simulink model "pwm1"  (R2012b)
settings: Solver=ode45  StartTime=0.0  StopTime=0.1  FixedStep=0.4e-4  RelTol=1e-3
libraries: Tools x5
settings Model: Creator=h3now  LastModifiedBy=h3now

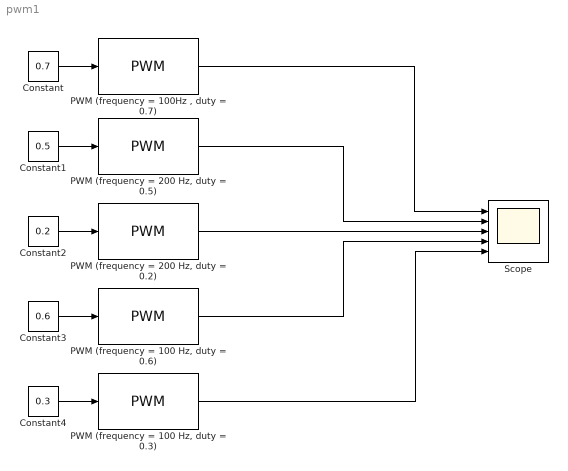
== system pwm1 ==
  Constant : Constant  Value=0.7
  Constant1 : Constant  Value=0.5
  Constant2 : Constant  Value=0.2
  Constant3 : Constant  Value=0.6
  Constant4 : Constant  Value=0.3
  "PWM (frequency = 100 Hz, duty = 0.3) " : Tools/PWM  f=100
  "PWM (frequency = 100 Hz, duty = 0.6) " : Tools/PWM  f=100
  "PWM (frequency = 100Hz , duty = 0.7) " : Tools/PWM  f=100
  "PWM (frequency = 200 Hz, duty = 0.2) " : Tools/PWM  f=200
  "PWM (frequency = 200 Hz, duty = 0.5) " : Tools/PWM  f=100
  Scope : Scope  NumInputPorts=5
      settings: YMin=-5~-5~-5~-5~-5  YMax=5~5~5~5~5
  wires:
  Constant/1 -> "PWM (frequency = 100Hz , duty = 0.7) "/1
  Constant1/1 -> "PWM (frequency = 200 Hz, duty = 0.5) "/1
  Constant2/1 -> "PWM (frequency = 200 Hz, duty = 0.2) "/1
  Constant3/1 -> "PWM (frequency = 100 Hz, duty = 0.6) "/1
  Constant4/1 -> "PWM (frequency = 100 Hz, duty = 0.3) "/1
  "PWM (frequency = 200 Hz, duty = 0.2) "/1 -> Scope/3
  "PWM (frequency = 100 Hz, duty = 0.6) "/1 -> Scope/4
  "PWM (frequency = 100 Hz, duty = 0.3) "/1 -> Scope/5
  "PWM (frequency = 100Hz , duty = 0.7) "/1 -> Scope/1
  "PWM (frequency = 200 Hz, duty = 0.5) "/1 -> Scope/2
